simulink subsystem "Fourier_Decomposition_AF"  (R2024b)
settings: Solver=VariableStepAuto  StartTime=0.0  StopTime=10.0  RelTol=1e-3
undefined symbols (not defined in the file or in its folder): settings
settings Model: Creator=phippold  LastModifiedBy=phippold

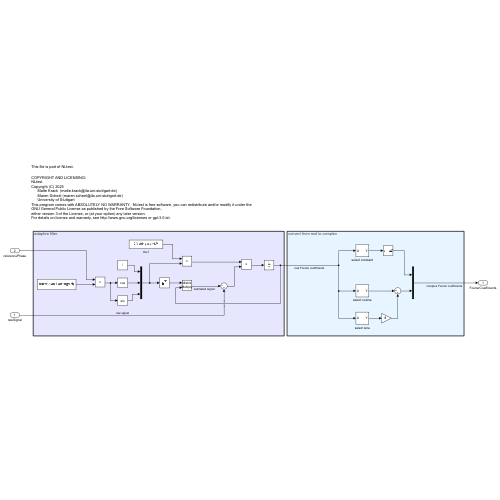
[thumbnail: Simulink's stored preview of the top-level diagram]
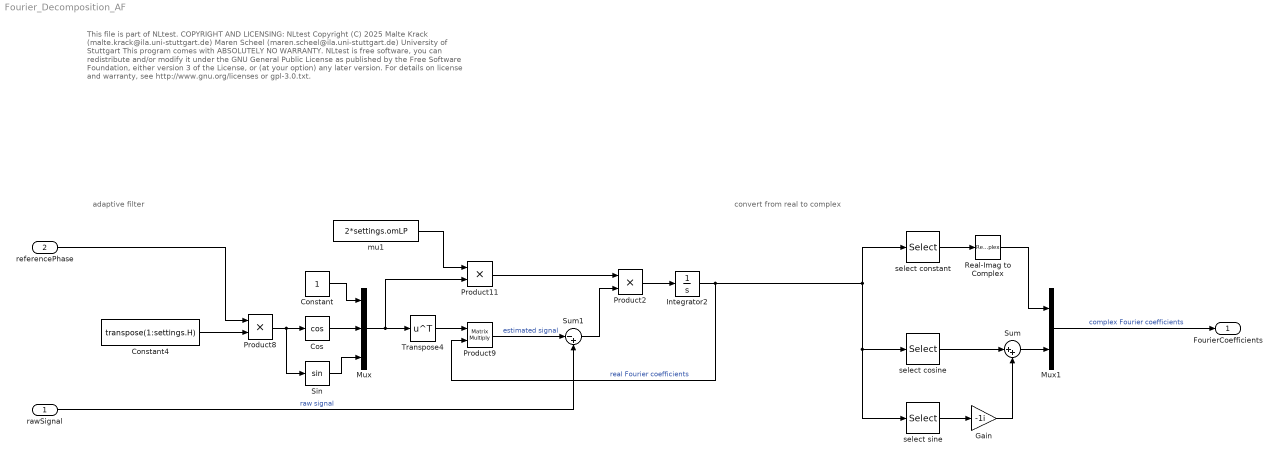
== system Fourier_Decomposition_AF ==
  note: convert from real to complex
  note: adaptive filter
  note: This file is part of NLtest.
      |
      | COPYRIGHT AND LICENSING:
      | NLtest
      | Copyright (C) 2025
      | Malte Krack (malte.krack@ila.uni-stuttgart.de)
      | Maren Scheel (maren.scheel@ila.uni-stuttgart.de)
      | University of Stuttgart
      | This program comes with ABSOLUTELY NO WARRANTY. NLtest is free software, you can redistribute and/or modify it under the GNU General Public License as published by the Free Software Foundation,
      | either version 3 of the License, or (at your option) any later version.
      | For details on license and warranty, see http://www.gnu.org/licenses or gpl-3.0.txt.
  rawSignal : Inport
  referencePhase : Inport  Port=2
  Constant : Constant
  Constant4 : Constant  Value=transpose(1:settings.H)  VectorParams1D=off
  Cos : Trigonometry  Operator=cos
  Gain : Gain  Gain=-1i
  Integrator2 : Integrator
  Mux : Mux  Inputs=3
  Mux1 : Mux  Inputs=2
  Product11 : Product
  Product2 : Product
  Product8 : Product
  Product9 : Product  Multiplication=Matrix(*)
  Real-Imag to Complex : RealImagToComplex  Input=Real
  Sin : Trigonometry
  Sum : Sum  Inputs=|++
  Sum1 : Sum  Inputs=|-+
  Transpose4 : Math  Operator=transpose  SignedPower=on
  mu1 : Constant  Value=2*settings.omLP
  select constant : Selector  InputPortWidth=2*settings.H+1  IndexOptions=Index vector (dialog)  Indices=1  OutputSizes=1
  select cosine : Selector  InputPortWidth=2*settings.H+1  IndexOptions=Index vector (dialog)  Indices=2:settings.H+1  OutputSizes=1
  select sine : Selector  InputPortWidth=2*settings.H+1  IndexOptions=Index vector (dialog)  Indices=settings.H+2:2*settings.H+1  OutputSizes=1
  FourierCoefficients : Outport
  wires:
  Integrator2/1 -> select constant/1, select sine/1, select cosine/1, Product9/2  "real Fourier coefficients"
  Sum1/1 -> Product2/2
  Product11/1 -> Product2/1
  Product2/1 -> Integrator2/1
  mu1/1 -> Product11/1
  Constant4/1 -> Product8/2
  Transpose4/1 -> Product9/1
  rawSignal/1 -> Sum1/2  "raw signal"
  referencePhase/1 -> Product8/1
  Mux/1 -> Transpose4/1, Product11/2
  Constant/1 -> Mux/1
  Sin/1 -> Mux/3
  Product8/1 -> Sin/1, Cos/1
  Cos/1 -> Mux/2
  Product9/1 -> Sum1/1  "estimated signal"
  select cosine/1 -> Sum/1
  select constant/1 -> Real-Imag to Complex/1
  select sine/1 -> Gain/1
  Sum/1 -> Mux1/2
  Gain/1 -> Sum/2
  Mux1/1 -> FourierCoefficients/1  "complex Fourier coefficients"
  Real-Imag to Complex/1 -> Mux1/1
